simulink model "assign_MBSD"  (R2019b)
settings: Solver=FixedStepDiscrete  StartTime=0.0  StopTime=inf  FixedStep=0.1  RelTol=1e-3  EnableMultiTasking=on
libraries: frdmk64flib x4, dspstat3 x3, simulink x3
settings Model: ExtModeTrigDuration=5  Creator=Cosimo  LastModifiedBy=Cosimo
settings OptimizationCC: EnhancedBackFolding=on  PassReuseOutputArgsAs=Individual arguments  ZeroExternalMemoryAtStartup=off  ZeroInternalMemoryAtStartup=off  MaxStackSize=64  OptimizeBlockOrder=speed  DifferentSizesBufferReuse=on  OptimizationCustomize=off  EfficientTunableParamExpr=on
settings DebuggingCC: ParameterTunabilityLossMsg=error
settings HardwareCC: ProdBitPerPointer=32  ProdBitPerSizeT=32  ProdBitPerPtrDiffT=32  ProdLargestAtomicInteger=Long  ProdLargestAtomicFloat=Double  ProdWordSize=32  ProdHWDeviceType=ARM Compatible->ARM Cortex
settings SFSimCC: MATLABDynamicMemAlloc=off
settings RTWCC: SystemTargetFile=ert.tlc  HardwareBoard=NXP FRDM-K64F  TLCOptions="-aInlineSetEventsForThisBaseRateFcn=TLC_FALSE -aSuppressMultiTaskScheduler=TLC_FALSE  -aRateBasedStepFcn=0"  TemplateMakefile=ert_default_tmf  GenerateReport=on  Toolchain=GNU Tools for ARM Embedded Processors  IncludeHyperlinkInReport=on  GenerateTraceInfo=on  GenerateTraceReport=on  GenerateTraceReportSl=on  GenerateTraceReportSf=on  GenerateTraceReportEml=on
settings CodeAppCC: ForceParamTrailComments=on  IgnoreCustomStorageClasses=off  OperatorAnnotations=on  SimulinkDataObjDesc=on  SFDataObjDesc=on  InsertBlockDesc=on

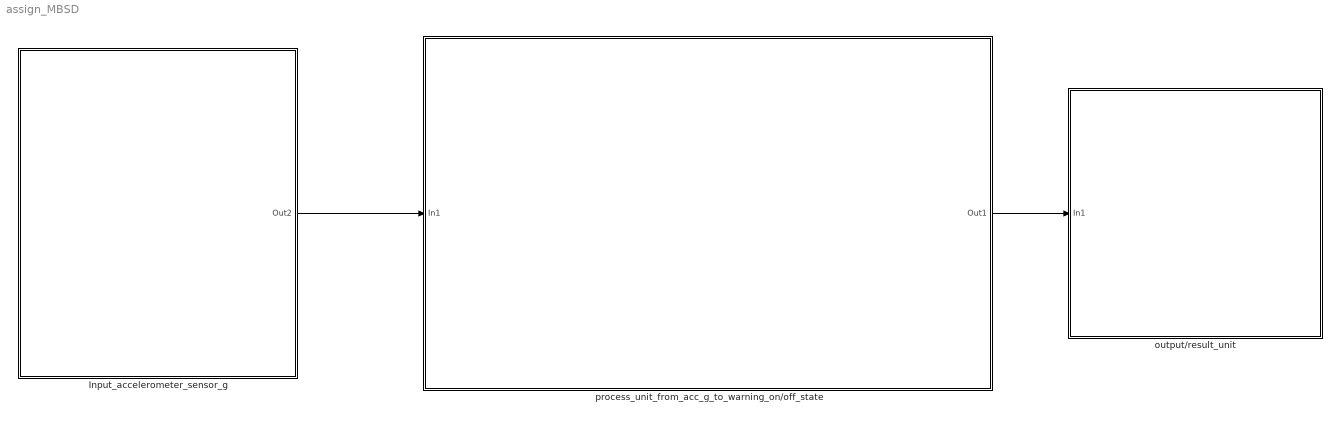
== system assign_MBSD ==
  Input_accelerometer_sensor_g : Subsystem
  output/result_unit : Subsystem
  process_unit_from_acc_g_to_warning_on/off_state : Subsystem
  wires:
  process_unit_from_acc_g_to_warning_on/off_state/1(Out1) -> output/result_unit/1(In1)
  Input_accelerometer_sensor_g/1(Out2) -> process_unit_from_acc_g_to_warning_on/off_state/1(In1)

== system assign_MBSD/Input_accelerometer_sensor_g ==
  note: FXOS8700CQ accellerometer block property of the board.
      | This block is the block to manage the acceleration of the axis of the board. The output is a triad of value [Acc_x,Acc_y,Acc_z] , in a range +2g / -2g
      | that will be managed by the next system.
  FXOS8700 6-Axes Sensor : frdmk64flib/FXOS8700 6-Axes Sensor  Activesensor=Accelerometer only  ODR=50Hz  HybridODR=400Hz  Accelfullrange=-2g to +2g  SampleTime=-1
      settings: SourceProductName=Simulink Coder Support Package for NXP FRDM-K64F Board
  Out2 : Outport
  wires:
  FXOS8700 6-Axes Sensor/1 -> Out2/1  "acc_on_three_axes_g"

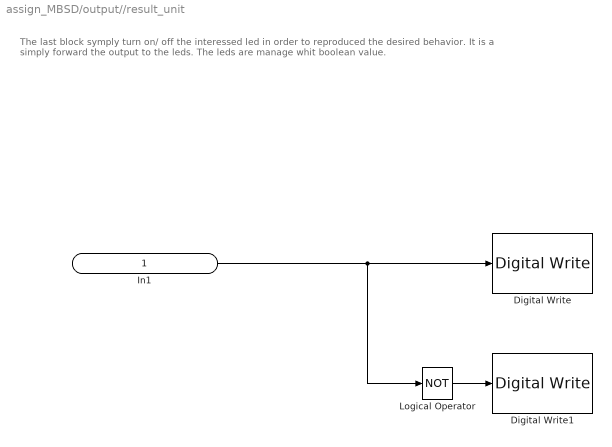
== system assign_MBSD/output//result_unit ==
  note: The last block symply turn on/ off the interessed led in order to reproduced the desired behavior.
      | It is a simply forward the output to the leds. The leds are manage whit boolean value.
  In1 : Inport
  Digital Write : frdmk64flib/Digital Write  Whichpin=RED_LED
      settings: SourceProductName=Simulink Coder Support Package for NXP FRDM-K64F Board
  Digital Write1 : frdmk64flib/Digital Write  Whichpin=GREEN_LED
      settings: SourceProductName=Simulink Coder Support Package for NXP FRDM-K64F Board
  Logical Operator : Logic  Operator=NOT  AllPortsSameDT=off  OutDataTypeStr=boolean
  wires:
  Logical Operator/1 -> Digital Write1/1
  In1/1 -> Logical Operator/1, Digital Write/1

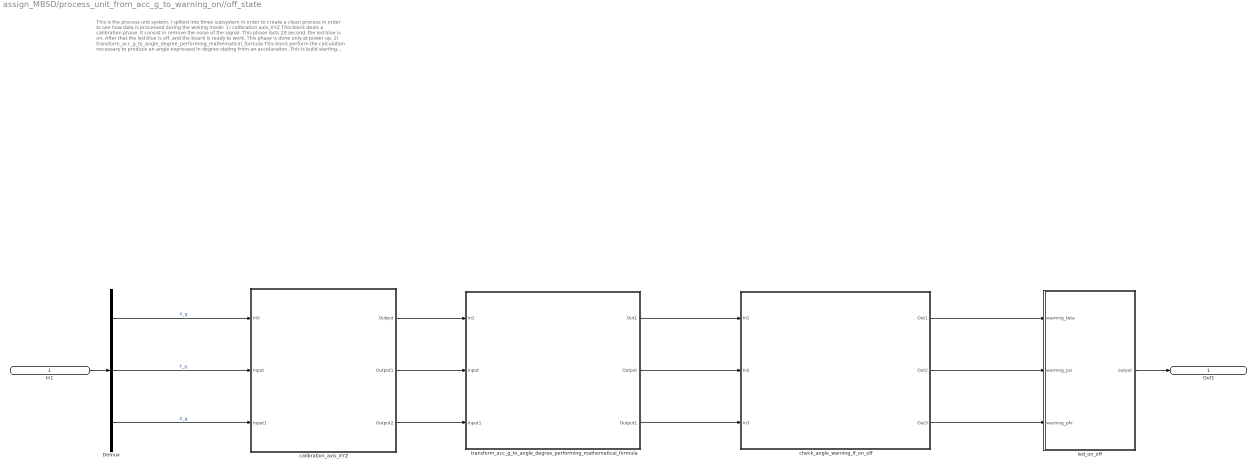
== system assign_MBSD/process_unit_from_acc_g_to_warning_on//off_state ==
  note: This is the process unit system.
      | I  splited into three subsystem in order to create a  clean process in order to see how data is processed during the woking mode:
      | 1) calibration axis_XYZ
      | 		This block deals a calibration phase. it consist in remove the noise of the signal. This phase lasts 20 second, the led blue is on. After that the led blue is off, and the board is ready to work.
      | 		This phase is done only at power up.
      |
      | 2) transform_acc_g_to_angle_degree_performing_mathematical_formula
      | 		This block perform the calculation necessary to produce an angle expressed in degree stating from an accelaration.
      | 		This is build starting from the forumula delivered on the pdf file. It is done just putting the simulink blok that model the operation needed
      |
      | 3)check_angle_warning_if_on_off
      | 		This block controll if the given input( angles)  is more than the threshold (15°) , or less than threshold.
      | 		This block perform also abosolute value of the signal , beacouse we are not  interested in sign o value of angle.
      |
      | 4) stateflow charts- led_on_off
      | 		This chatrs deals the on/off led ( red and green ) . In input receive variable that assume only two values(0,1), 0 on variable means no error on that angle, 1 waring on that angle
      | 		Red: warning if one of axis does not respect the threshold
      | 		Green: if no warning is raised.
      |
      |
      | The integration test of this system is done considering that when we moving the board there are correation between the axis.
      | The acceleration detected by the x-axis is proportional to the sine of the angle of inclination.
      | The y-axis acceleration, due to the orthogonality, is proportional to the sine + phase ( cosine)  of the angle of inclination.
      | The z-axis acceleration, due to the orthogonality on the x-y plane, is proportional to the sine   of the angle of inclination
      |
      | Each subsystem have more than one test harness in order to model the behavoir of the system concern.
  In1 : Inport
  Demux : Demux  Outputs=3
  calibration_axis_XYZ : Subsystem
  check_angle_warning_if_on_off : Subsystem
  "led_on_off " : Stateflow chart  BlockKeywords=__PRM__SERIALIZED__DATA__:Stateflow Chart,Stateflow Diagram  TreatAsAtomicUnit=on
  "transform_acc_g_to_angle_degree_performing_mathematical_formula " : Subsystem
  Out1 : Outport
  wires:
  check_angle_warning_if_on_off/2(Out2) -> "led_on_off "/2(warning_psi)
  check_angle_warning_if_on_off/1(Out1) -> "led_on_off "/1(warning_teta)
  "transform_acc_g_to_angle_degree_performing_mathematical_formula "/2(Output) -> check_angle_warning_if_on_off/2(In2)
  check_angle_warning_if_on_off/3(Out3) -> "led_on_off "/3(warning_phi)
  "transform_acc_g_to_angle_degree_performing_mathematical_formula "/1(Out1) -> check_angle_warning_if_on_off/1(In1)
  "transform_acc_g_to_angle_degree_performing_mathematical_formula "/3(Output1) -> check_angle_warning_if_on_off/3(In3)
  "led_on_off "/1(output) -> Out1/1
  Demux/2 -> calibration_axis_XYZ/2(Input)  "Y_g"
  Demux/1 -> calibration_axis_XYZ/1(In5)  "X_g"
  calibration_axis_XYZ/2(Output1) -> "transform_acc_g_to_angle_degree_performing_mathematical_formula "/2(Input)
  calibration_axis_XYZ/3(Output2) -> "transform_acc_g_to_angle_degree_performing_mathematical_formula "/3(Input1)
  Demux/3 -> calibration_axis_XYZ/3(Input1)  "Z_g"
  calibration_axis_XYZ/1(Output) -> "transform_acc_g_to_angle_degree_performing_mathematical_formula "/1(In1)
  In1/1 -> Demux/1

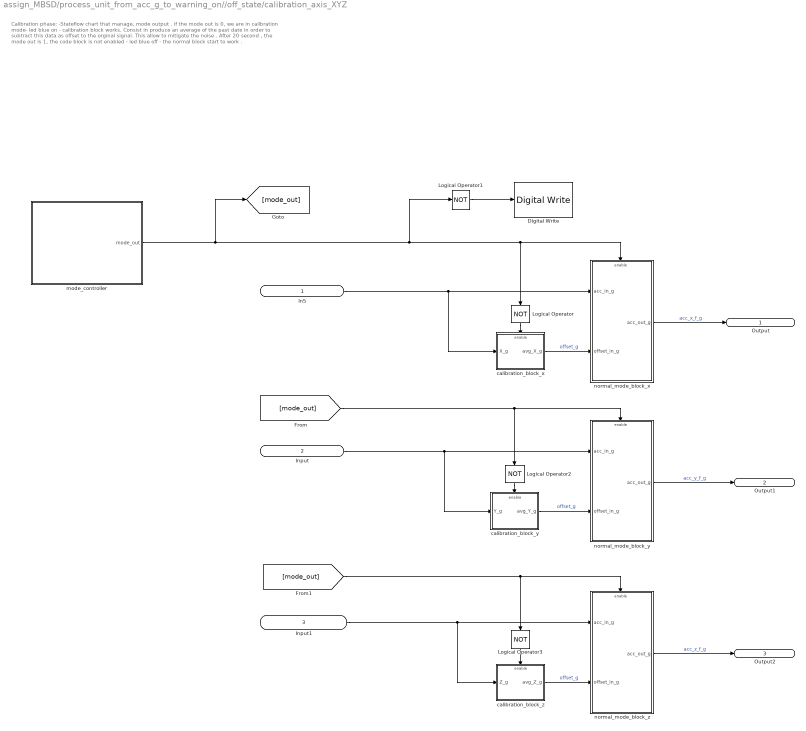
== system assign_MBSD/process_unit_from_acc_g_to_warning_on//off_state/calibration_axis_XYZ ==
  note: Calibration phase:
      |
      | -Stateflow chart that manage, mode output .
      | 	if the mode out is 0, we are in calibration mode- led blue on - calibration block works. Consist in produce an average of the past date in order to subtract this data as offset to the orginal signal.
      | 	This allow to mitigate the noise .
      | 	After 20 second , the mode out is 1, the code block is not enabled -  led blue off  - the normal block start to work .
  In5 : Inport
  Input : Inport  Port=2
  Input1 : Inport  Port=3
  Digital Write : frdmk64flib/Digital Write  Whichpin=BLUE_LED
      settings: SourceProductName=Simulink Coder Support Package for NXP FRDM-K64F Board
  Logical Operator{,1..3} (4 alike) : Logic  Operator=NOT  AllPortsSameDT=off  OutDataTypeStr=boolean
  calibration_block_x : Subsystem
  calibration_block_y : Subsystem
  calibration_block_z : Subsystem
  mode_controller : Stateflow chart  BlockKeywords=__PRM__SERIALIZED__DATA__:Stateflow Chart,Stateflow Diagram  TreatAsAtomicUnit=on
  normal_mode_block_x : Subsystem
  normal_mode_block_y : Subsystem
  normal_mode_block_z : Subsystem
  Output : Outport
  Output1 : Outport  Port=2
  Output2 : Outport  Port=3
  wires:
  normal_mode_block_y/1(acc_out_g) -> Output1/1  "acc_y_f_g"
  [mode_out] -> Logical Operator3/1, normal_mode_block_z/Enable
  calibration_block_z/1(avg_Z_g) -> normal_mode_block_z/2(offset_in_g)  "offset_g"
  Input1/1 -> calibration_block_z/1(Z_g), normal_mode_block_z/1(acc_in_g)
  [mode_out] -> normal_mode_block_y/Enable, Logical Operator2/1
  calibration_block_y/1(avg_Y_g) -> normal_mode_block_y/2(offset_in_g)  "offset_g"
  Input/1 -> calibration_block_y/1(Y_g), normal_mode_block_y/1(acc_in_g)
  normal_mode_block_x/1(acc_out_g) -> Output/1  "acc_x_f_g"
  Logical Operator1/1 -> Digital Write/1
  calibration_block_x/1(avg_X_g) -> normal_mode_block_x/2(offset_in_g)  "offset_g"
  mode_controller/1(mode_out) -> Logical Operator/1, normal_mode_block_x/Enable, Logical Operator1/1, [mode_out]
  In5/1 -> normal_mode_block_x/1(acc_in_g), calibration_block_x/1(X_g)
  Logical Operator/1 -> calibration_block_x/Enable
  Logical Operator2/1 -> calibration_block_y/Enable
  Logical Operator3/1 -> calibration_block_z/Enable
  normal_mode_block_z/1(acc_out_g) -> Output2/1  "acc_z_f_g"

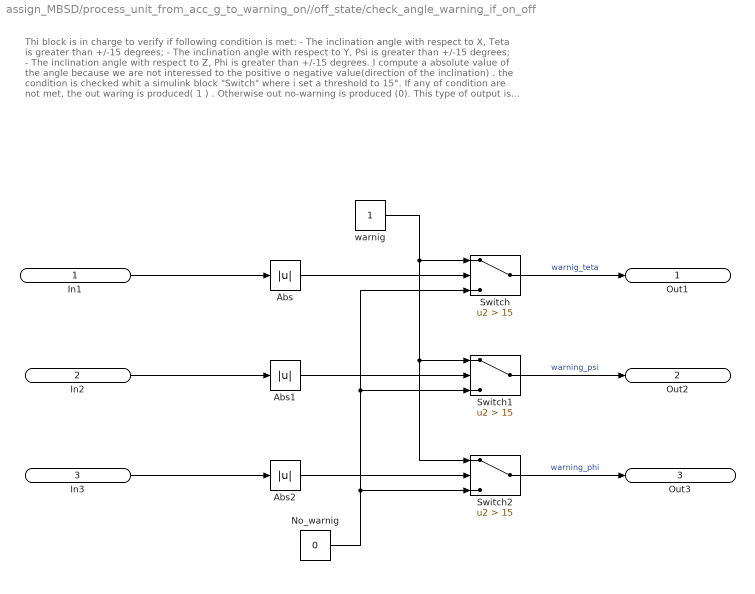
== system assign_MBSD/process_unit_from_acc_g_to_warning_on//off_state/check_angle_warning_if_on_off ==
  note: Thi block is in charge to verify if following condition is met:
      | - The inclination angle with respect to  X, Teta is greater than +/-15 degrees;
      | - The inclination angle with respect to  Y,  Psi is greater than +/-15 degrees;
      | - The inclination angle with respect to  Z,  Phi is greater than +/-15 degrees.
      |
      | I compute a absolute value of the angle because we are not interessed to the positive o negative value(direction of the inclination) .
      |
      | the condition is checked whit a simulink block "Switch" where i set a threshold to 15°.
      | If any of condition are not met, the out waring is produced( 1 ) . Otherwise out no-warning is produced (0). This type of output is useful for the stateflow system
  In1 : Inport
  In2 : Inport  Port=2
  In3 : Inport  Port=3
  Abs : Abs
  Abs1 : Abs
  Abs2 : Abs
  No_warnig : Constant  Value=0
  Switch : Switch  Criteria=u2 > Threshold  Threshold=15
  Switch1 : Switch  Criteria=u2 > Threshold  Threshold=15
  Switch2 : Switch  Criteria=u2 > Threshold  Threshold=15
  "warnig " : Constant
  Out1 : Outport
  Out2 : Outport  Port=2
  Out3 : Outport  Port=3
  wires:
  "warnig "/1 -> Switch2/1, Switch1/1, Switch/1
  No_warnig/1 -> Switch2/3, Switch1/3, Switch/3
  In2/1 -> Abs1/1
  In3/1 -> Abs2/1
  Abs2/1 -> Switch2/2
  Abs1/1 -> Switch1/2
  In1/1 -> Abs/1
  Abs/1 -> Switch/2
  Switch2/1 -> Out3/1  "warning_phi"
  Switch1/1 -> Out2/1  "warning_psi"
  Switch/1 -> Out1/1  "warnig_teta"

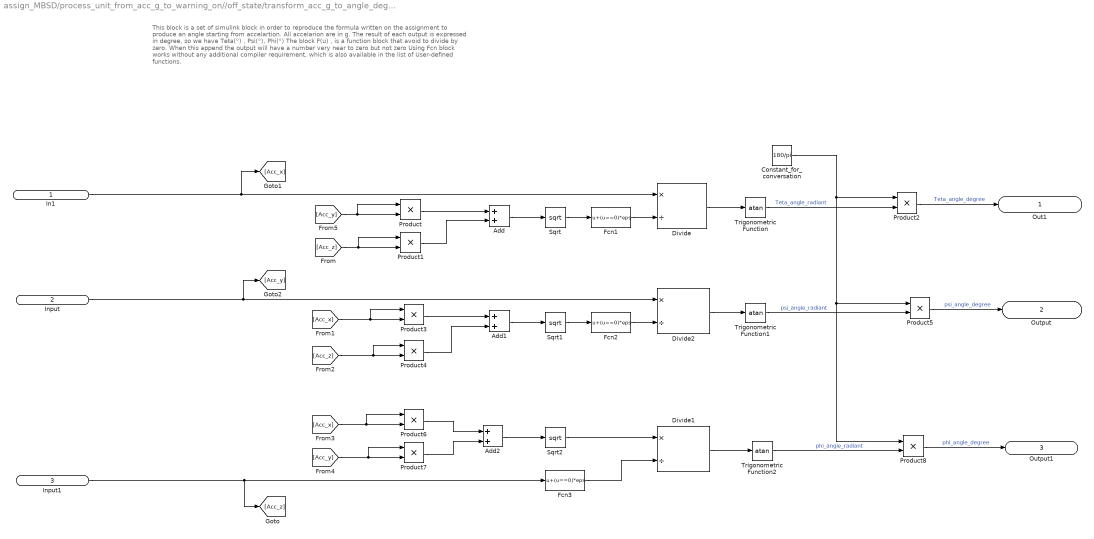
== system assign_MBSD/process_unit_from_acc_g_to_warning_on//off_state/transform_acc_g_to_angle_degree_performing_mathematical_formula  ==
  note: This block is a set of simulink block in order to reproduce the formula written on the assignment to produce an angle starting
      | from accelartion.
      | All accelarion are in g.
      | The result of each output is expressed in degree, so we have Teta(°) , Psi(°), Phi(°)
      |
      | The block F(u) , is a function block that avoid to divide by zero. When this append the output will have a number very near to zero but not zero
      | Using Fcn block  works without any additional compiler requirement, which is also available in the list of User-defined functions.
  In1 : Inport
  Input : Inport  Port=2
  Input1 : Inport  Port=3
  Add : Sum
  Add1 : Sum
  Add2 : Sum
  Constant_for_conversation : Constant  Value=180/pi
  Divide : Product  Inputs=*/
  Divide1 : Product  Inputs=*/
  Divide2 : Product  Inputs=*/
  Fcn1 : Fcn  Expr=u+(u==0)*eps
  Fcn2 : Fcn  Expr=u+(u==0)*eps
  Fcn3 : Fcn  Expr=u+(u==0)*eps
  Product{,1..8} (9 alike) : Product
  Sqrt : Sqrt  SaturateOnIntegerOverflow=on
  Sqrt1 : Sqrt  SaturateOnIntegerOverflow=on
  Sqrt2 : Sqrt  SaturateOnIntegerOverflow=on
  Trigonometric Function : Trigonometry  Operator=atan
  Trigonometric Function1 : Trigonometry  Operator=atan
  Trigonometric Function2 : Trigonometry  Operator=atan
  Out1 : Outport
  Output : Outport  Port=2
  Output1 : Outport  Port=3
  wires:
  Add/1 -> Sqrt/1
  Product/1 -> Add/1
  Product1/1 -> Add/2
  Sqrt/1 -> Fcn1/1
  Product2/1 -> Out1/1  "Teta_angle_degree"
  Trigonometric Function/1 -> Product2/2  "Teta_angle_radiant"
  Constant_for_conversation/1 -> Product8/1, Product5/1, Product2/1
  [Acc_z] -> Product1/1, Product1/2
  Sqrt1/1 -> Fcn2/1
  Add1/1 -> Sqrt1/1
  [Acc_x] -> Product3/1, Product3/2
  Product3/1 -> Add1/1
  [Acc_z] -> Product4/1, Product4/2
  Product4/1 -> Add1/2
  Trigonometric Function1/1 -> Product5/2  "psi_angle_radiant"
  Product5/1 -> Output/1  "psi_angle_degree"
  Divide2/1 -> Trigonometric Function1/1
  Sqrt2/1 -> Divide1/1
  Add2/1 -> Sqrt2/1
  Product6/1 -> Add2/1
  Product7/1 -> Add2/2
  [Acc_x] -> Product6/1, Product6/2
  [Acc_y] -> Product7/2, Product7/1
  Divide1/1 -> Trigonometric Function2/1
  Trigonometric Function2/1 -> Product8/2  "phi_angle_radiant"
  Product8/1 -> Output1/1  "phi_angle_degree"
  [Acc_y] -> Product/1, Product/2
  Divide/1 -> Trigonometric Function/1
  Fcn1/1 -> Divide/2
  Fcn2/1 -> Divide2/2
  Fcn3/1 -> Divide1/2
  In1/1 -> Divide/1, [Acc_x]
  Input/1 -> Divide2/1, [Acc_y]
  Input1/1 -> [Acc_z], Fcn3/1

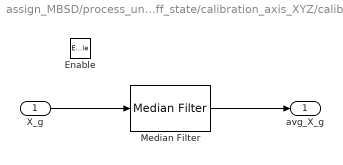
== system assign_MBSD/process_unit_from_acc_g_to_warning_on//off_state/calibration_axis_XYZ/calibration_block_x ==
  X_g : Inport
  Enable : EnablePort
  Median Filter : dspstat3/Median Filter  WindowLength=128  SimulateUsing=Code generation
      settings: SourceProductName=DSP System Toolbox  SourceProductBaseCode=DS
  avg_X_g : Outport
  wires:
  Median Filter/1 -> avg_X_g/1
  X_g/1 -> Median Filter/1

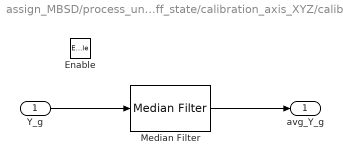
== system assign_MBSD/process_unit_from_acc_g_to_warning_on//off_state/calibration_axis_XYZ/calibration_block_y ==
  Y_g : Inport
  Enable : EnablePort
  Median Filter : dspstat3/Median Filter  WindowLength=128  SimulateUsing=Code generation
      settings: SourceProductName=DSP System Toolbox  SourceProductBaseCode=DS
  avg_Y_g : Outport
  wires:
  Y_g/1 -> Median Filter/1
  Median Filter/1 -> avg_Y_g/1

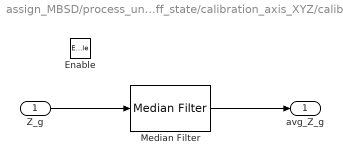
== system assign_MBSD/process_unit_from_acc_g_to_warning_on//off_state/calibration_axis_XYZ/calibration_block_z ==
  Z_g : Inport
  Enable : EnablePort
  Median Filter : dspstat3/Median Filter  WindowLength=128  SimulateUsing=Code generation
      settings: SourceProductName=DSP System Toolbox  SourceProductBaseCode=DS
  avg_Z_g : Outport
  wires:
  Median Filter/1 -> avg_Z_g/1
  Z_g/1 -> Median Filter/1

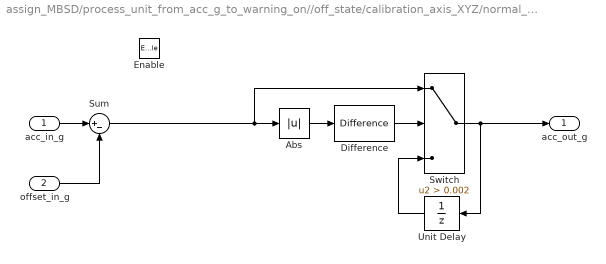
== system assign_MBSD/process_unit_from_acc_g_to_warning_on//off_state/calibration_axis_XYZ/normal_mode_block_x ==
  acc_in_g : Inport
  offset_in_g : Inport  Port=2
  Enable : EnablePort
  Abs : Abs
  Difference : simulink/Discrete/Difference  ICPrevInput=0.0  OutMin=[]  OutMax=[]  OutDataType=fixdt(1, 16)  OutScaling=2^-10  DoSatur=off
  Sum : Sum  Inputs=|+-
  Switch : Switch  Criteria=u2 > Threshold  Threshold=0.002
  Unit Delay : UnitDelay  SampleTime=-1  HasFrameUpgradeWarning=on
  acc_out_g : Outport
  wires:
  offset_in_g/1 -> Sum/2
  acc_in_g/1 -> Sum/1
  Unit Delay/1 -> Switch/3
  Abs/1 -> Difference/1
  Switch/1 -> acc_out_g/1, Unit Delay/1
  Difference/1 -> Switch/2
  Sum/1 -> Switch/1, Abs/1

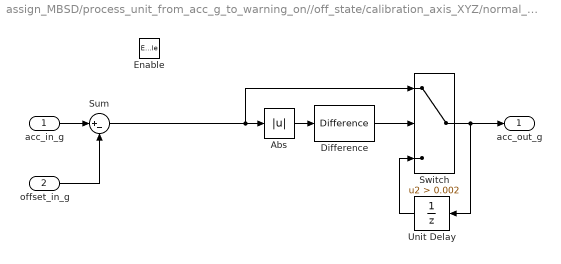
== system assign_MBSD/process_unit_from_acc_g_to_warning_on//off_state/calibration_axis_XYZ/normal_mode_block_y ==
  acc_in_g : Inport
  offset_in_g : Inport  Port=2
  Enable : EnablePort
  Abs : Abs
  Difference : simulink/Discrete/Difference  ICPrevInput=0.0  OutMin=[]  OutMax=[]  OutDataType=fixdt(1, 16)  OutScaling=2^-10  DoSatur=off
  Sum : Sum  Inputs=|+-
  Switch : Switch  Criteria=u2 > Threshold  Threshold=0.002
  Unit Delay : UnitDelay  SampleTime=-1  HasFrameUpgradeWarning=on
  acc_out_g : Outport
  wires:
  acc_in_g/1 -> Sum/1
  offset_in_g/1 -> Sum/2
  Unit Delay/1 -> Switch/3
  Abs/1 -> Difference/1
  Switch/1 -> acc_out_g/1, Unit Delay/1
  Difference/1 -> Switch/2
  Sum/1 -> Switch/1, Abs/1

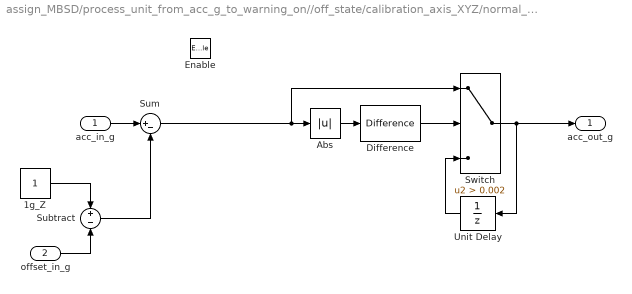
== system assign_MBSD/process_unit_from_acc_g_to_warning_on//off_state/calibration_axis_XYZ/normal_mode_block_z ==
  acc_in_g : Inport
  offset_in_g : Inport  Port=2
  Enable : EnablePort
  1g_Z : Constant  SampleTime=-1
  Abs : Abs
  Difference : simulink/Discrete/Difference  ICPrevInput=0.0  OutMin=[]  OutMax=[]  OutDataType=fixdt(1, 16)  OutScaling=2^-10  DoSatur=off
  Subtract : Sum  Inputs=+-
  Sum : Sum  Inputs=|+-
  Switch : Switch  Criteria=u2 > Threshold  Threshold=0.002
  Unit Delay : UnitDelay  SampleTime=-1  HasFrameUpgradeWarning=on
  acc_out_g : Outport
  wires:
  acc_in_g/1 -> Sum/1
  Unit Delay/1 -> Switch/3
  Abs/1 -> Difference/1
  Switch/1 -> acc_out_g/1, Unit Delay/1
  Difference/1 -> Switch/2
  Sum/1 -> Switch/1, Abs/1
  1g_Z/1 -> Subtract/1
  offset_in_g/1 -> Subtract/2
  Subtract/1 -> Sum/2

== stateflow chart assign_MBSD/process_unit_from_acc_g_to_warning_on//off_state/calibration_axis_XYZ/mode_controller ==
  state calibration_state
    en:
    mode_out=0;
  state normal_state
    en:
    mode_out=1;
  (default) -> calibration_state
  calibration_state -> normal_state : after(20,sec)
  data: mode_out output int8

== stateflow chart assign_MBSD/process_unit_from_acc_g_to_warning_on//off_state/led_on_off  ==
  note: Stateflow chart that manage when activate a Red Led or Green Led, This is done by cheking the value o warning each time. This Value
      | Is given by input to the chart.
  state state_no_error
    en:
    output=0;
  state state_error
    en:
    output=1;
  (default) -> state_no_error
  state_error -> state_no_error : [[warning_teta==0 && warning_psi==0 && warning_phi==0]]
  state_no_error -> state_error : [warning_teta==1 || warning_psi==1 || warning_phi==1]
  data: warning_teta input; warning_psi input; warning_phi input; output output
